simulink model "first_princ_controller_try"  (R2021a)
settings: Solver=VariableStepAuto  StartTime=0.0  StopTime=2500  RelTol=1e-3
libraries: pid_lib x4
(part 2 of 2)

== system first_princ_controller_try/Subsystem9 ==
  Del Hr1 : Constant  Value=3.56*10^5
  Divide{1..4,6..7} (6 alike) : Product  Inputs=*/
  Divide5 : Product  Inputs=/*
  If1 : Constant  Value=7632.2
  Integrator3 : Integrator  InitialCondition=7632.2
  Integrator4 : Integrator  InitialCondition=587.47
  Integrator5 : Integrator  InitialCondition=415
  Integrator6 : Integrator  InitialCondition=326
  Kd1 : Gain  Gain=8.86*10^-20
  Kp1 : Gain  Gain=0.193
  Mf1 : Constant  Value=587.47
  Ot2 : Gain  Gain=6.13
  P1 : Constant  Value=8.25*10^-6
  Product10 : Product  Inputs=3
  Product{2,5..6,9,11..12} (6 alike) : Product
  Qc1 : Gain  Gain=0.251
  Qi1 : Constant  Value=6.13
  Qm1 : Constant  Value=6.13
  Qt1 : Gain  Gain=6.13
  Qt3 : Gain  Gain=6.13
  Row Cp1 : Constant  Value=4.184*10^3*858.085
  Row c Cpc1 : Constant  Value=4.184*10^3*858.085
  Scope : Scope
  Step : Step  Time=0  SampleTime=0
  Sum1 : Sum  Inputs=|++
  Sum10 : Sum  Inputs=|++-
  Sum{8,11,13,16} (4 alike) : Sum  Inputs=|-+
  Sum12 : Sum  Inputs=|+-
  Sum14 : Sum  Inputs=|++
  Sum15 : Sum  Inputs=|+-
  Sum17 : Sum  Inputs=|+-
  Tcf1 : Constant  Value=326
  Tf1 : Constant  Value=415
  V1 : Constant  Value=14.07
  Vc1 : Constant  Value=0.4919
  hA1 : Constant  Value=3842.37
  wires:
  Qm1/1 -> Product5/1
  Sum12/1 -> Product9/1
  Sum10/1 -> Integrator5/1
  Integrator5/1 -> Scope/1, Sum12/1, Sum11/1  "TR"
  Ot2/1 -> Sum16/1
  Product11/1 -> Divide5/1
  Divide4/1 -> Sum10/2
  Sum16/1 -> Divide2/1
  Del Hr1/1 -> Product10/1
  Qi1/1 -> Product2/1
  Divide5/1 -> Sum10/3
  hA1/1 -> Product9/2
  Row c Cpc1/1 -> Product12/2
  Product10/1 -> Divide4/1
  Kd1/1 -> Sum15/2
  If1/1 -> Product2/2
  Divide3/1 -> Sum10/1
  Product6/1 -> Sum17/2
  Mf1/1 -> Product5/2
  Sum17/1 -> Integrator4/1
  Qt1/1 -> Sum8/1
  Kp1/1 -> Product6/1, Product10/2  "Kp"
  Tcf1/1 -> Sum13/2
  Integrator3/1 -> Kd1/1, Qt1/1  "M"
  Product9/1 -> Divide5/2, Divide7/1  "T hA(T-Tc)"
  Row Cp1/1 -> Product11/2, Divide4/2
  Sum11/1 -> Qt3/1
  Divide1/1 -> Sum15/1
  Product5/1 -> Sum16/2
  P1/1 -> Product6/2, Product10/3  "P"
  Vc1/1 -> Product12/1, Divide6/2
  Product2/1 -> Sum8/2
  V1/1 -> Product11/1, Divide3/2, Divide2/2, Divide1/2  "V"
  Sum8/1 -> Divide1/1
  Integrator4/1 -> Kp1/1, Ot2/1  "S"
  Divide6/1 -> Sum14/1
  Divide2/1 -> Sum17/1
  Divide7/1 -> Sum14/2
  Tf1/1 -> Sum11/2
  Qc1/1 -> Divide6/1
  Sum13/1 -> Qc1/1
  Product12/1 -> Divide7/2
  Integrator6/1 -> Sum13/1, Sum12/2  "TC"
  Qt3/1 -> Divide3/1
  Sum14/1 -> Integrator6/1
  Sum1/1 -> Integrator3/1
  Sum15/1 -> Sum1/2
  Step/1 -> Sum1/1
